simulink library "speedgoatlib_evse"  (R2024b)
settings: Solver=VariableStepAuto  StartTime=0.0  StopTime=10.0  RelTol=1e-3
undefined symbols (not defined in the file): sg_ev_charging_read_m, sg_ev_charging_write_m, sg_ev_isolation_read_m, sg_ev_parameter_read_m, sg_ev_parameter_write_m, sg_ev_precharge_read_m, sg_ev_precharge_write_m, sg_ev_status_m, sg_ev_stop_read_m, sg_ev_stop_write_m, sg_ev_welding_read_m, sg_ev_welding_write_m, sg_evse_charging_read_m, sg_evse_charging_write_m, sg_evse_isolation_read_m, sg_evse_isolation_write_m, sg_evse_parameter_read_m, sg_evse_parameter_write_m, sg_evse_precharge_read_m, sg_evse_precharge_write_m, sg_evse_status_m, sg_evse_stop_read_m, sg_evse_stop_write_m, sg_evse_welding_read_m, sg_evse_welding_write_m
libraries: speedgoatlib_mqtt x199, simulink x39, $bdroot x24
(part 5 of 8)

== system speedgoatlib_evse/Blocks by Charge State/EV Welding Read /string compare logic1 ==
  Input : Inport
  ASCII to String1 : ASCIIToString
  Add : Sum
  Gain : Gain  Gain=2
  String Compare : StringCompare
  String Compare1 : StringCompare
  String Constant : StringConstant  String="\"started\""
  String Constant1 : StringConstant  String="\"finished\""
  Out1 : Outport
  wires:
  Input/1 -> ASCII to String1/1
  Add/1 -> Out1/1
  Gain/1 -> Add/2
  String Compare1/1 -> Gain/1
  String Constant/1 -> String Compare/2
  String Compare/1 -> Add/1
  String Constant1/1 -> String Compare1/2
  ASCII to String1/1 -> String Compare/1, String Compare1/1

== system speedgoatlib_evse/Blocks by Charge State/EV Welding Write /Enabled Subsystem ==
  ready : Inport
  errorcode : Inport  Port=2
  resssoc : Inport  Port=3
  Enable : EnablePort
  Constant1 : Constant  Value=parEnErrorCode  OutDataTypeStr=boolean
  Constant2 : Constant  Value=parEnRessSoc  OutDataTypeStr=boolean
  Constant5 : Constant  Value=parEnReady  OutDataTypeStr=boolean
  Data Type Conversion1 : DataTypeConversion  OutDataTypeStr=double  SaturateOnIntegerOverflow=off  RndMeth=Floor
  Ground1 : Ground
  Ground2 : Ground
  Ground5 : Ground
  String to ASCII1 : StringToASCII  OutputVectorSize=12
  String to ASCII2 : StringToASCII  OutputVectorSize=12
  String to ASCII3 : StringToASCII  OutputVectorSize=24
  To String1 : ToString
  To String2 : ToString
  To String3 : ToString
  port0_ci_ev_welding_errorcode : speedgoatlib_mqtt/Client/MQTT Client Publish  ClientId=parClientId  ConnectionId=parConnectionId  Topic='port0/ci/ev/welding/errorcode'  QoS=0 - at most once  Retain=on  Extended=on  SampleTime=parSampleTime
      settings: SourceProductName=MQTT
  port0_ci_ev_welding_ready : speedgoatlib_mqtt/Client/MQTT Client Publish  ClientId=parClientId  ConnectionId=parConnectionId  Topic='port0/ci/ev/welding/ready'  QoS=0 - at most once  Retain=on  Extended=on  SampleTime=parSampleTime
      settings: SourceProductName=MQTT
  port0_ci_ev_welding_resssoc : speedgoatlib_mqtt/Client/MQTT Client Publish  ClientId=parClientId  ConnectionId=parConnectionId  Topic='port0/ci/ev/welding/resssoc'  QoS=0 - at most once  Retain=on  Extended=on  SampleTime=parSampleTime
      settings: SourceProductName=MQTT
  wires:
  ready/1 -> Data Type Conversion1/1
  To String1/1 -> String to ASCII1/1
  String to ASCII1/1 -> port0_ci_ev_welding_ready/1
  String to ASCII2/1 -> port0_ci_ev_welding_resssoc/1
  To String2/1 -> String to ASCII2/1
  resssoc/1 -> To String2/1
  Data Type Conversion1/1 -> To String1/1
  To String3/1 -> String to ASCII3/1
  errorcode/1 -> To String3/1
  String to ASCII3/1 -> port0_ci_ev_welding_errorcode/1
  Constant5/1 -> port0_ci_ev_welding_ready/2
  Ground5/1 -> port0_ci_ev_welding_ready/3
  Ground1/1 -> port0_ci_ev_welding_errorcode/3
  Constant1/1 -> port0_ci_ev_welding_errorcode/2
  Constant2/1 -> port0_ci_ev_welding_resssoc/2
  Ground2/1 -> port0_ci_ev_welding_resssoc/3

== system speedgoatlib_evse/Blocks by Charge State/EV Welding Write /string compare logic ==
  Input : Inport
  ASCII to String1 : ASCIIToString
  Add : Sum
  Gain : Gain  Gain=2
  String Compare : StringCompare
  String Compare1 : StringCompare
  String Constant : StringConstant  String="\"started\""
  String Constant1 : StringConstant  String="\"finished\""
  Out1 : Outport
  wires:
  ASCII to String1/1 -> String Compare1/1, String Compare/1
  String Constant1/1 -> String Compare1/2
  String Compare/1 -> Add/1
  String Constant/1 -> String Compare/2
  String Compare1/1 -> Gain/1
  Gain/1 -> Add/2
  Add/1 -> Out1/1
  Input/1 -> ASCII to String1/1

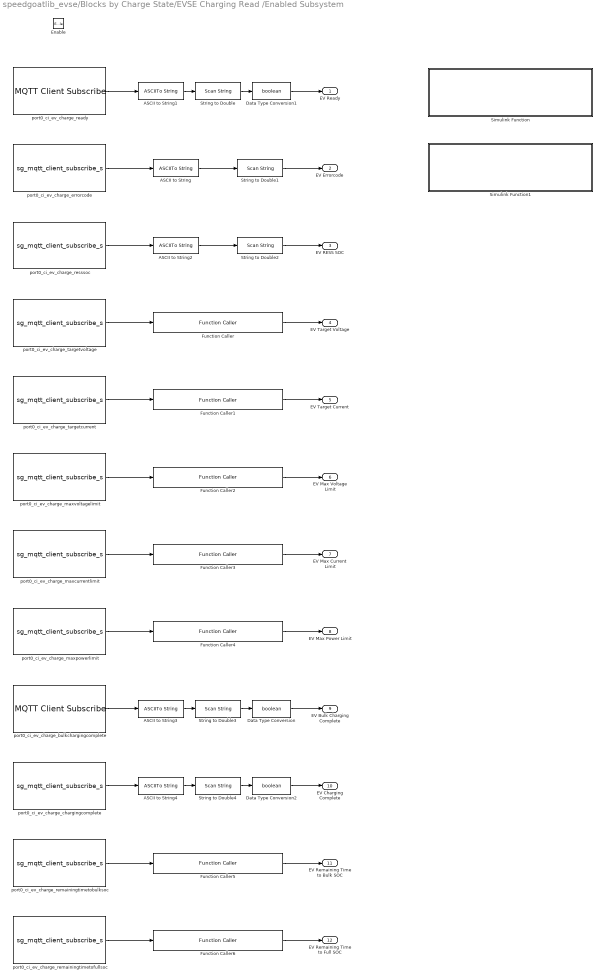
== system speedgoatlib_evse/Blocks by Charge State/EVSE Charging Read /Enabled Subsystem ==
  Enable : EnablePort
  ASCII to String{,1..4} (5 alike) : ASCIIToString
  Data Type Conversion : DataTypeConversion  OutDataTypeStr=boolean  SaturateOnIntegerOverflow=off  RndMeth=Floor
  Data Type Conversion1 : DataTypeConversion  OutDataTypeStr=boolean  SaturateOnIntegerOverflow=off  RndMeth=Floor
  Data Type Conversion2 : DataTypeConversion  OutDataTypeStr=boolean  SaturateOnIntegerOverflow=off  RndMeth=Floor
  Function Caller{,1..4} (5 alike) : FunctionCaller  FunctionPrototype=value = fromJsonPhysicalValue(uint8_vec)  InputArgumentSpecifications=zeros(1,48,'uint8')  OutputArgumentSpecifications=double(0)
  Function Caller5 : FunctionCaller  FunctionPrototype=value = fromJsonPhysicalValueUnit(uint8_vec)  InputArgumentSpecifications=zeros(1,64,'uint8')  OutputArgumentSpecifications=double(0)
  Function Caller6 : FunctionCaller  FunctionPrototype=value = fromJsonPhysicalValueUnit(uint8_vec)  InputArgumentSpecifications=zeros(1,64,'uint8')  OutputArgumentSpecifications=double(0)
  Simulink Function : Subsystem  TreatAsAtomicUnit=on
  Simulink Function1 : Subsystem  TreatAsAtomicUnit=on
  String to Double{,1..4} (5 alike) : ScanString  Format="\"%lf\""
  port0_ci_ev_charge_bulkchargingcomplete : speedgoatlib_mqtt/Client/MQTT Client Subscribe  ClientId=parClientId  ConnectionId=parConnectionId  Topic='port0/ci/ev/charge/bulkchargingcomplete'  QoS=0 - at most once  InitValue=zeros(1,12,'uint8')  Extended=off  SampleTime=parSampleTime
      settings: SourceProductName=MQTT
  port0_ci_ev_charge_chargingcomplete : S-Function  FunctionName=sg_mqtt_client_subscribe_s  Parameters="ClientId,  ConnectionId, Topic, QoS, InitValue, Extended, SampleTime"  SFunctionDeploymentMode=off  EnableBusSupport=off  mask(mqtt_client_subscribe_1){ClientId=parClientId, ConnectionId=parConnectionId, Topic='port0/ci/ev/charge/chargingcomplete', QoS=0 - at most once, InitValue=zeros(1,12,'uint8'), Extended=off, SampleTime=parSampleTime}
      mask prompts: ClientId "Station ID"; ConnectionId "Connection ID"; QoS "Quality of Service"; InitValue "Init Value"; Extended "Extended Interface"; SampleTime "Sample Time [s]"
      mask help: Speedgoat Driver Block<br>MQTT Client - Subscribe<br><br>&copy; 2007 - 2023, Speedgoat GmbH, <a href="matlab: web('www.speedgoat.com','-browser');">www.speedgoat.com</a>
      mask init:
      | sg_mqtt_client_subscribe_m.runMaskInitialization(ClientId, ConnectionId, Topic, InitValue, Extended);
      mask Help: eval('sg.utils.help.show(''io_main/refentry_mqtt_client_subscribe'');')
      mask TypeOptions QoS: 0 - at most once | 1 - at least once | 2 - exactly once
      mask DialogControl groupParameters Prompt: Parameters
      mask Display: disp('Speedgoat\nMQTT Client\nSubscribe\nStation ID: 0\nConnection ID: 0');
  port0_ci_ev_charge_errorcode : S-Function  FunctionName=sg_mqtt_client_subscribe_s  Parameters="ClientId,  ConnectionId, Topic, QoS, InitValue, Extended, SampleTime"  SFunctionDeploymentMode=off  EnableBusSupport=off  mask(mqtt_client_subscribe_1){ClientId=parClientId, ConnectionId=parConnectionId, Topic='port0/ci/ev/charge/errorcode', QoS=0 - at most once, InitValue=zeros(1,24,'uint8'), Extended=off, SampleTime=parSampleTime}
      mask prompts: ClientId "Station ID"; ConnectionId "Connection ID"; QoS "Quality of Service"; InitValue "Init Value"; Extended "Extended Interface"; SampleTime "Sample Time [s]"
      mask help: Speedgoat Driver Block<br>MQTT Client - Subscribe<br><br>&copy; 2007 - 2023, Speedgoat GmbH, <a href="matlab: web('www.speedgoat.com','-browser');">www.speedgoat.com</a>
      mask init:
      | sg_mqtt_client_subscribe_m.runMaskInitialization(ClientId, ConnectionId, Topic, InitValue, Extended);
      mask Help: eval('sg.utils.help.show(''io_main/refentry_mqtt_client_subscribe'');')
      mask TypeOptions QoS: 0 - at most once | 1 - at least once | 2 - exactly once
      mask DialogControl groupParameters Prompt: Parameters
      mask Display: disp('Speedgoat\nMQTT Client\nSubscribe\nStation ID: 0\nConnection ID: 0');
  port0_ci_ev_charge_maxcurrentlimit : S-Function  FunctionName=sg_mqtt_client_subscribe_s  Parameters="ClientId,  ConnectionId, Topic, QoS, InitValue, Extended, SampleTime"  SFunctionDeploymentMode=off  EnableBusSupport=off  mask(mqtt_client_subscribe_1){ClientId=parClientId, ConnectionId=parConnectionId, Topic='port0/ci/ev/charge/maxcurrentlimit', QoS=0 - at most once, InitValue=zeros(1,48,'uint8'), Extended=off, SampleTime=parSampleTime}
      mask prompts: ClientId "Station ID"; ConnectionId "Connection ID"; QoS "Quality of Service"; InitValue "Init Value"; Extended "Extended Interface"; SampleTime "Sample Time [s]"
      mask help: Speedgoat Driver Block<br>MQTT Client - Subscribe<br><br>&copy; 2007 - 2023, Speedgoat GmbH, <a href="matlab: web('www.speedgoat.com','-browser');">www.speedgoat.com</a>
      mask init:
      | sg_mqtt_client_subscribe_m.runMaskInitialization(ClientId, ConnectionId, Topic, InitValue, Extended);
      mask Help: eval('sg.utils.help.show(''io_main/refentry_mqtt_client_subscribe'');')
      mask TypeOptions QoS: 0 - at most once | 1 - at least once | 2 - exactly once
      mask DialogControl groupParameters Prompt: Parameters
      mask Display: disp('Speedgoat\nMQTT Client\nSubscribe\nStation ID: 0\nConnection ID: 0');
  port0_ci_ev_charge_maxpowerlimit : S-Function  FunctionName=sg_mqtt_client_subscribe_s  Parameters="ClientId,  ConnectionId, Topic, QoS, InitValue, Extended, SampleTime"  SFunctionDeploymentMode=off  EnableBusSupport=off  mask(mqtt_client_subscribe_1){ClientId=parClientId, ConnectionId=parConnectionId, Topic='port0/ci/ev/charge/maxpowerlimit', QoS=0 - at most once, InitValue=zeros(1,48,'uint8'), Extended=off, SampleTime=parSampleTime}
      mask prompts: ClientId "Station ID"; ConnectionId "Connection ID"; QoS "Quality of Service"; InitValue "Init Value"; Extended "Extended Interface"; SampleTime "Sample Time [s]"
      mask help: Speedgoat Driver Block<br>MQTT Client - Subscribe<br><br>&copy; 2007 - 2023, Speedgoat GmbH, <a href="matlab: web('www.speedgoat.com','-browser');">www.speedgoat.com</a>
      mask init:
      | sg_mqtt_client_subscribe_m.runMaskInitialization(ClientId, ConnectionId, Topic, InitValue, Extended);
      mask Help: eval('sg.utils.help.show(''io_main/refentry_mqtt_client_subscribe'');')
      mask TypeOptions QoS: 0 - at most once | 1 - at least once | 2 - exactly once
      mask DialogControl groupParameters Prompt: Parameters
      mask Display: disp('Speedgoat\nMQTT Client\nSubscribe\nStation ID: 0\nConnection ID: 0');
  port0_ci_ev_charge_maxvoltagelimit : S-Function  FunctionName=sg_mqtt_client_subscribe_s  Parameters="ClientId,  ConnectionId, Topic, QoS, InitValue, Extended, SampleTime"  SFunctionDeploymentMode=off  EnableBusSupport=off  mask(mqtt_client_subscribe_1){ClientId=parClientId, ConnectionId=parConnectionId, Topic='port0/ci/ev/charge/maxvoltagelimit', QoS=0 - at most once, InitValue=zeros(1,48,'uint8'), Extended=off, SampleTime=parSampleTime}
      mask prompts: ClientId "Station ID"; ConnectionId "Connection ID"; QoS "Quality of Service"; InitValue "Init Value"; Extended "Extended Interface"; SampleTime "Sample Time [s]"
      mask help: Speedgoat Driver Block<br>MQTT Client - Subscribe<br><br>&copy; 2007 - 2023, Speedgoat GmbH, <a href="matlab: web('www.speedgoat.com','-browser');">www.speedgoat.com</a>
      mask init:
      | sg_mqtt_client_subscribe_m.runMaskInitialization(ClientId, ConnectionId, Topic, InitValue, Extended);
      mask Help: eval('sg.utils.help.show(''io_main/refentry_mqtt_client_subscribe'');')
      mask TypeOptions QoS: 0 - at most once | 1 - at least once | 2 - exactly once
      mask DialogControl groupParameters Prompt: Parameters
      mask Display: disp('Speedgoat\nMQTT Client\nSubscribe\nStation ID: 0\nConnection ID: 0');
  port0_ci_ev_charge_ready : speedgoatlib_mqtt/Client/MQTT Client Subscribe  ClientId=parClientId  ConnectionId=parConnectionId  Topic='port0/ci/ev/charge/ready'  QoS=0 - at most once  InitValue=zeros(1,12,'uint8')  Extended=off  SampleTime=parSampleTime
      settings: SourceProductName=MQTT
  port0_ci_ev_charge_remainingtimetobulksoc : S-Function  FunctionName=sg_mqtt_client_subscribe_s  Parameters="ClientId,  ConnectionId, Topic, QoS, InitValue, Extended, SampleTime"  SFunctionDeploymentMode=off  EnableBusSupport=off  mask(mqtt_client_subscribe_1){ClientId=parClientId, ConnectionId=parConnectionId, Topic='port0/ci/ev/charge/remainingtimetobulksoc', QoS=0 - at most once, InitValue=zeros(1,64,'uint8'), Extended=off, SampleTime=parSampleTime}
      mask prompts: ClientId "Station ID"; ConnectionId "Connection ID"; QoS "Quality of Service"; InitValue "Init Value"; Extended "Extended Interface"; SampleTime "Sample Time [s]"
      mask help: Speedgoat Driver Block<br>MQTT Client - Subscribe<br><br>&copy; 2007 - 2023, Speedgoat GmbH, <a href="matlab: web('www.speedgoat.com','-browser');">www.speedgoat.com</a>
      mask init:
      | sg_mqtt_client_subscribe_m.runMaskInitialization(ClientId, ConnectionId, Topic, InitValue, Extended);
      mask Help: eval('sg.utils.help.show(''io_main/refentry_mqtt_client_subscribe'');')
      mask TypeOptions QoS: 0 - at most once | 1 - at least once | 2 - exactly once
      mask DialogControl groupParameters Prompt: Parameters
      mask Display: disp('Speedgoat\nMQTT Client\nSubscribe\nStation ID: 0\nConnection ID: 0');
  port0_ci_ev_charge_remainingtimetofullsoc : S-Function  FunctionName=sg_mqtt_client_subscribe_s  Parameters="ClientId,  ConnectionId, Topic, QoS, InitValue, Extended, SampleTime"  SFunctionDeploymentMode=off  EnableBusSupport=off  mask(mqtt_client_subscribe_1){ClientId=parClientId, ConnectionId=parConnectionId, Topic='port0/ci/ev/charge/remainingtimetofullsoc', QoS=0 - at most once, InitValue=zeros(1,64,'uint8'), Extended=off, SampleTime=parSampleTime}
      mask prompts: ClientId "Station ID"; ConnectionId "Connection ID"; QoS "Quality of Service"; InitValue "Init Value"; Extended "Extended Interface"; SampleTime "Sample Time [s]"
      mask help: Speedgoat Driver Block<br>MQTT Client - Subscribe<br><br>&copy; 2007 - 2023, Speedgoat GmbH, <a href="matlab: web('www.speedgoat.com','-browser');">www.speedgoat.com</a>
      mask init:
      | sg_mqtt_client_subscribe_m.runMaskInitialization(ClientId, ConnectionId, Topic, InitValue, Extended);
      mask Help: eval('sg.utils.help.show(''io_main/refentry_mqtt_client_subscribe'');')
      mask TypeOptions QoS: 0 - at most once | 1 - at least once | 2 - exactly once
      mask DialogControl groupParameters Prompt: Parameters
      mask Display: disp('Speedgoat\nMQTT Client\nSubscribe\nStation ID: 0\nConnection ID: 0');
  port0_ci_ev_charge_resssoc : S-Function  FunctionName=sg_mqtt_client_subscribe_s  Parameters="ClientId,  ConnectionId, Topic, QoS, InitValue, Extended, SampleTime"  SFunctionDeploymentMode=off  EnableBusSupport=off  mask(mqtt_client_subscribe_1){ClientId=parClientId, ConnectionId=parConnectionId, Topic='port0/ci/ev/charge/resssoc', QoS=0 - at most once, InitValue=zeros(1,12,'uint8'), Extended=off, SampleTime=parSampleTime}
      mask prompts: ClientId "Station ID"; ConnectionId "Connection ID"; QoS "Quality of Service"; InitValue "Init Value"; Extended "Extended Interface"; SampleTime "Sample Time [s]"
      mask help: Speedgoat Driver Block<br>MQTT Client - Subscribe<br><br>&copy; 2007 - 2023, Speedgoat GmbH, <a href="matlab: web('www.speedgoat.com','-browser');">www.speedgoat.com</a>
      mask init:
      | sg_mqtt_client_subscribe_m.runMaskInitialization(ClientId, ConnectionId, Topic, InitValue, Extended);
      mask Help: eval('sg.utils.help.show(''io_main/refentry_mqtt_client_subscribe'');')
      mask TypeOptions QoS: 0 - at most once | 1 - at least once | 2 - exactly once
      mask DialogControl groupParameters Prompt: Parameters
      mask Display: disp('Speedgoat\nMQTT Client\nSubscribe\nStation ID: 0\nConnection ID: 0');
  port0_ci_ev_charge_targetcurrent : S-Function  FunctionName=sg_mqtt_client_subscribe_s  Parameters="ClientId,  ConnectionId, Topic, QoS, InitValue, Extended, SampleTime"  SFunctionDeploymentMode=off  EnableBusSupport=off  mask(mqtt_client_subscribe_1){ClientId=parClientId, ConnectionId=parConnectionId, Topic='port0/ci/ev/charge/targetcurrent', QoS=0 - at most once, InitValue=zeros(1,48,'uint8'), Extended=off, SampleTime=parSampleTime}
      mask prompts: ClientId "Station ID"; ConnectionId "Connection ID"; QoS "Quality of Service"; InitValue "Init Value"; Extended "Extended Interface"; SampleTime "Sample Time [s]"
      mask help: Speedgoat Driver Block<br>MQTT Client - Subscribe<br><br>&copy; 2007 - 2023, Speedgoat GmbH, <a href="matlab: web('www.speedgoat.com','-browser');">www.speedgoat.com</a>
      mask init:
      | sg_mqtt_client_subscribe_m.runMaskInitialization(ClientId, ConnectionId, Topic, InitValue, Extended);
      mask Help: eval('sg.utils.help.show(''io_main/refentry_mqtt_client_subscribe'');')
      mask TypeOptions QoS: 0 - at most once | 1 - at least once | 2 - exactly once
      mask DialogControl groupParameters Prompt: Parameters
      mask Display: disp('Speedgoat\nMQTT Client\nSubscribe\nStation ID: 0\nConnection ID: 0');
  port0_ci_ev_charge_targetvoltage : S-Function  FunctionName=sg_mqtt_client_subscribe_s  Parameters="ClientId,  ConnectionId, Topic, QoS, InitValue, Extended, SampleTime"  SFunctionDeploymentMode=off  EnableBusSupport=off  mask(mqtt_client_subscribe_1){ClientId=parClientId, ConnectionId=parConnectionId, Topic='port0/ci/ev/charge/targetvoltage', QoS=0 - at most once, InitValue=zeros(1,48,'uint8'), Extended=off, SampleTime=parSampleTime}
      mask prompts: ClientId "Station ID"; ConnectionId "Connection ID"; QoS "Quality of Service"; InitValue "Init Value"; Extended "Extended Interface"; SampleTime "Sample Time [s]"
      mask help: Speedgoat Driver Block<br>MQTT Client - Subscribe<br><br>&copy; 2007 - 2023, Speedgoat GmbH, <a href="matlab: web('www.speedgoat.com','-browser');">www.speedgoat.com</a>
      mask init:
      | sg_mqtt_client_subscribe_m.runMaskInitialization(ClientId, ConnectionId, Topic, InitValue, Extended);
      mask Help: eval('sg.utils.help.show(''io_main/refentry_mqtt_client_subscribe'');')
      mask TypeOptions QoS: 0 - at most once | 1 - at least once | 2 - exactly once
      mask DialogControl groupParameters Prompt: Parameters
      mask Display: disp('Speedgoat\nMQTT Client\nSubscribe\nStation ID: 0\nConnection ID: 0');
  EV Ready : Outport
  EV Errorcode : Outport  Port=2
  EV RESS SOC : Outport  Port=3
  EV Target Voltage : Outport  Port=4
  EV Target Current : Outport  Port=5
  EV Max Voltage Limit : Outport  Port=6
  EV Max Current Limit : Outport  Port=7
  EV Max Power Limit : Outport  Port=8
  EV Bulk Charging Complete : Outport  Port=9
  EV Charging Complete : Outport  Port=10
  EV Remaining Time to Bulk SOC : Outport  Port=11
  EV Remaining Time to Full SOC : Outport  Port=12
  wires:
  port0_ci_ev_charge_ready/1 -> ASCII to String1/1
  port0_ci_ev_charge_errorcode/1 -> ASCII to String/1
  ASCII to String/1 -> String to Double1/1
  ASCII to String1/1 -> String to Double/1
  String to Double/1 -> Data Type Conversion1/1
  String to Double1/1 -> EV Errorcode/1
  String to Double2/1 -> EV RESS SOC/1
  ASCII to String2/1 -> String to Double2/1
  port0_ci_ev_charge_resssoc/1 -> ASCII to String2/1
  Function Caller/1 -> EV Target Voltage/1
  port0_ci_ev_charge_targetvoltage/1 -> Function Caller/1
  port0_ci_ev_charge_targetcurrent/1 -> Function Caller1/1
  Function Caller1/1 -> EV Target Current/1
  Function Caller2/1 -> EV Max Voltage Limit/1
  port0_ci_ev_charge_maxvoltagelimit/1 -> Function Caller2/1
  port0_ci_ev_charge_maxcurrentlimit/1 -> Function Caller3/1
  Function Caller3/1 -> EV Max Current Limit/1
  Function Caller4/1 -> EV Max Power Limit/1
  port0_ci_ev_charge_maxpowerlimit/1 -> Function Caller4/1
  String to Double3/1 -> Data Type Conversion/1
  ASCII to String3/1 -> String to Double3/1
  port0_ci_ev_charge_bulkchargingcomplete/1 -> ASCII to String3/1
  Data Type Conversion/1 -> EV Bulk Charging Complete/1
  Data Type Conversion1/1 -> EV Ready/1
  Data Type Conversion2/1 -> EV Charging Complete/1
  port0_ci_ev_charge_chargingcomplete/1 -> ASCII to String4/1
  ASCII to String4/1 -> String to Double4/1
  String to Double4/1 -> Data Type Conversion2/1
  port0_ci_ev_charge_remainingtimetobulksoc/1 -> Function Caller5/1
  Function Caller5/1 -> EV Remaining Time to Bulk SOC/1
  Function Caller6/1 -> EV Remaining Time to Full SOC/1
  port0_ci_ev_charge_remainingtimetofullsoc/1 -> Function Caller6/1

== system speedgoatlib_evse/Blocks by Charge State/EVSE Charging Read /string compare logic ==
  Input : Inport
  ASCII to String1 : ASCIIToString
  Add : Sum
  Gain : Gain  Gain=2
  String Compare : StringCompare
  String Compare1 : StringCompare
  String Constant : StringConstant  String="\"started\""
  String Constant1 : StringConstant  String="\"finished\""
  Out1 : Outport
  wires:
  Input/1 -> ASCII to String1/1
  Add/1 -> Out1/1
  Gain/1 -> Add/2
  String Compare1/1 -> Gain/1
  String Constant/1 -> String Compare/2
  String Compare/1 -> Add/1
  String Constant1/1 -> String Compare1/2
  ASCII to String1/1 -> String Compare/1, String Compare1/1

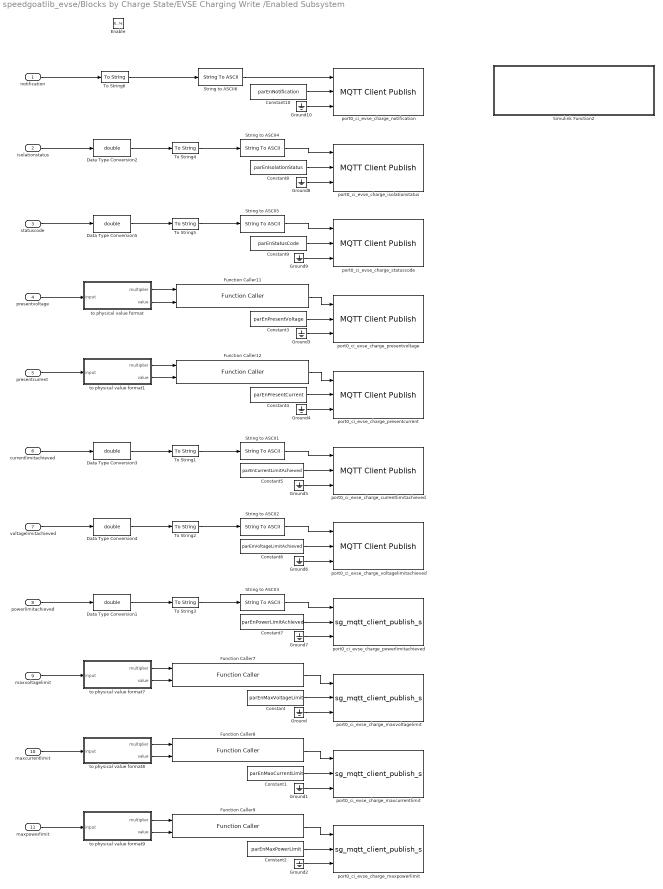
== system speedgoatlib_evse/Blocks by Charge State/EVSE Charging Write /Enabled Subsystem ==
  notification : Inport
  isolationstatus : Inport  Port=2
  statuscode : Inport  Port=3
  presentvoltage : Inport  Port=4
  presentcurrent : Inport  Port=5
  currentlimitachieved : Inport  Port=6
  voltagelimitachieved : Inport  Port=7
  powerlimitachieved : Inport  Port=8
  maxvoltagelimit : Inport  Port=9
  maxcurrentlimit : Inport  Port=10
  maxpowerlimit : Inport  Port=11
  Enable : EnablePort
  Constant : Constant  Value=parEnMaxVoltageLimit  OutDataTypeStr=boolean
  Constant1 : Constant  Value=parEnMaxCurrentLimit  OutDataTypeStr=boolean
  Constant10 : Constant  Value=parEnNotification  OutDataTypeStr=boolean
  Constant2 : Constant  Value=parEnMaxPowerLimit  OutDataTypeStr=boolean
  Constant3 : Constant  Value=parEnPresentVoltage  OutDataTypeStr=boolean
  Constant4 : Constant  Value=parEnPresentCurrent  OutDataTypeStr=boolean
  Constant5 : Constant  Value=parEnCurrentLimitAchieved  OutDataTypeStr=boolean
  Constant6 : Constant  Value=parEnVoltageLimitAchieved  OutDataTypeStr=boolean
  Constant7 : Constant  Value=parEnPowerLimitAchieved  OutDataTypeStr=boolean
  Constant8 : Constant  Value=parEnIsolationStatus  OutDataTypeStr=boolean
  Constant9 : Constant  Value=parEnStatusCode  OutDataTypeStr=boolean
  Data Type Conversion{1..5} (5 alike) : DataTypeConversion  OutDataTypeStr=double  SaturateOnIntegerOverflow=off  RndMeth=Floor
  Function Caller{7..9,11..12} (5 alike) : FunctionCaller  FunctionPrototype=json_string = toJsonPhysicalValue(multiplier,value)  InputArgumentSpecifications=double(0), double(0)  OutputArgumentSpecifications=zeros(1,48,'uint8')
  Ground{,1..10} (11 alike) : Ground
  Simulink Function2 : Subsystem  TreatAsAtomicUnit=on
  String to ASCII{1..5} (5 alike) : StringToASCII  OutputVectorSize=12
  String to ASCII6 : StringToASCII  OutputVectorSize=16
  To String{1..6} (6 alike) : ToString
  port0_ci_evse_charge_currentlimitachieved : speedgoatlib_mqtt/Client/MQTT Client Publish  ClientId=parClientId  ConnectionId=parConnectionId  Topic='port0/ci/evse/charge/currentlimitachieved'  QoS=0 - at most once  Retain=on  Extended=on  SampleTime=parSampleTime
      settings: SourceProductName=MQTT
  port0_ci_evse_charge_isolationstatus : speedgoatlib_mqtt/Client/MQTT Client Publish  ClientId=parClientId  ConnectionId=parConnectionId  Topic='port0/ci/evse/charge/isolationstatus'  QoS=0 - at most once  Retain=on  Extended=on  SampleTime=parSampleTime
      settings: SourceProductName=MQTT
  port0_ci_evse_charge_maxcurrentlimit : S-Function  FunctionName=sg_mqtt_client_publish_s  Parameters="ClientId,  ConnectionId, Topic, QoS, Retain, Extended, SampleTime"  SFunctionDeploymentMode=off  EnableBusSupport=off  mask(mqtt_client_publish_1){ClientId=parClientId, ConnectionId=parConnectionId, Topic='port0/ci/evse/charge/maxcurrentlimit', QoS=0 - at most once, Retain=on, Extended=on, SampleTime=parSampleTime}
      mask prompts: ClientId "Station ID"; ConnectionId "Connection ID"; QoS "Quality of Service"; Extended "Extended Interface"; SampleTime "Sample Time [s]"
      mask help: Speedgoat Driver Block<br>MQTT Client - Publish<br><br>&copy; 2007 - 2023, Speedgoat GmbH, <a href="matlab: web('www.speedgoat.com','-browser');">www.speedgoat.com</a>
      mask init:
      | sg_mqtt_client_publish_m.runMaskInitialization(ClientId, ConnectionId, Topic, Extended);
      mask Help: eval('sg.utils.help.show(''io_main/refentry_mqtt_client_publish'');')
      mask TypeOptions QoS: 0 - at most once | 1 - at least once | 2 - exactly once
      mask DialogControl groupParameters Prompt: Parameters
      mask Display: text(0.9,0.5,'Speedgoat\nMQTT Client\nPublish\nStation ID: 0\nConnection ID: 0','horizontalAlignment', 'right','verticalAlignment', 'middle');port_label('input',1,'Data');port_label('input',2,'Enable');port_label('input',3,'Length');
  port0_ci_evse_charge_maxpowerlimit : S-Function  FunctionName=sg_mqtt_client_publish_s  Parameters="ClientId,  ConnectionId, Topic, QoS, Retain, Extended, SampleTime"  SFunctionDeploymentMode=off  EnableBusSupport=off  mask(mqtt_client_publish_1){ClientId=parClientId, ConnectionId=parConnectionId, Topic='port0/ci/evse/charge/maxpowerlimit', QoS=0 - at most once, Retain=on, Extended=on, SampleTime=parSampleTime}
      mask prompts: ClientId "Station ID"; ConnectionId "Connection ID"; QoS "Quality of Service"; Extended "Extended Interface"; SampleTime "Sample Time [s]"
      mask help: Speedgoat Driver Block<br>MQTT Client - Publish<br><br>&copy; 2007 - 2023, Speedgoat GmbH, <a href="matlab: web('www.speedgoat.com','-browser');">www.speedgoat.com</a>
      mask init:
      | sg_mqtt_client_publish_m.runMaskInitialization(ClientId, ConnectionId, Topic, Extended);
      mask Help: eval('sg.utils.help.show(''io_main/refentry_mqtt_client_publish'');')
      mask TypeOptions QoS: 0 - at most once | 1 - at least once | 2 - exactly once
      mask DialogControl groupParameters Prompt: Parameters
      mask Display: text(0.9,0.5,'Speedgoat\nMQTT Client\nPublish\nStation ID: 0\nConnection ID: 0','horizontalAlignment', 'right','verticalAlignment', 'middle');port_label('input',1,'Data');port_label('input',2,'Enable');port_label('input',3,'Length');
  port0_ci_evse_charge_maxvoltagelimit : S-Function  FunctionName=sg_mqtt_client_publish_s  Parameters="ClientId,  ConnectionId, Topic, QoS, Retain, Extended, SampleTime"  SFunctionDeploymentMode=off  EnableBusSupport=off  mask(mqtt_client_publish_1){ClientId=parClientId, ConnectionId=parConnectionId, Topic='port0/ci/evse/charge/maxvoltagelimit', QoS=0 - at most once, Retain=on, Extended=on, SampleTime=parSampleTime}
      mask prompts: ClientId "Station ID"; ConnectionId "Connection ID"; QoS "Quality of Service"; Extended "Extended Interface"; SampleTime "Sample Time [s]"
      mask help: Speedgoat Driver Block<br>MQTT Client - Publish<br><br>&copy; 2007 - 2023, Speedgoat GmbH, <a href="matlab: web('www.speedgoat.com','-browser');">www.speedgoat.com</a>
      mask init:
      | sg_mqtt_client_publish_m.runMaskInitialization(ClientId, ConnectionId, Topic, Extended);
      mask Help: eval('sg.utils.help.show(''io_main/refentry_mqtt_client_publish'');')
      mask TypeOptions QoS: 0 - at most once | 1 - at least once | 2 - exactly once
      mask DialogControl groupParameters Prompt: Parameters
      mask Display: text(0.9,0.5,'Speedgoat\nMQTT Client\nPublish\nStation ID: 0\nConnection ID: 0','horizontalAlignment', 'right','verticalAlignment', 'middle');port_label('input',1,'Data');port_label('input',2,'Enable');port_label('input',3,'Length');
  port0_ci_evse_charge_notification : speedgoatlib_mqtt/Client/MQTT Client Publish  ClientId=parClientId  ConnectionId=parConnectionId  Topic='port0/ci/evse/charge/notification'  QoS=0 - at most once  Retain=on  Extended=on  SampleTime=parSampleTime
      settings: SourceProductName=MQTT
  port0_ci_evse_charge_powerlimitachieved : S-Function  FunctionName=sg_mqtt_client_publish_s  Parameters="ClientId,  ConnectionId, Topic, QoS, Retain, Extended, SampleTime"  SFunctionDeploymentMode=off  EnableBusSupport=off  mask(mqtt_client_publish_1){ClientId=parClientId, ConnectionId=parConnectionId, Topic='port0/ci/evse/charge/powerlimitachieved', QoS=0 - at most once, Retain=on, Extended=on, SampleTime=parSampleTime}
      mask prompts: ClientId "Station ID"; ConnectionId "Connection ID"; QoS "Quality of Service"; Extended "Extended Interface"; SampleTime "Sample Time [s]"
      mask help: Speedgoat Driver Block<br>MQTT Client - Publish<br><br>&copy; 2007 - 2023, Speedgoat GmbH, <a href="matlab: web('www.speedgoat.com','-browser');">www.speedgoat.com</a>
      mask init:
      | sg_mqtt_client_publish_m.runMaskInitialization(ClientId, ConnectionId, Topic, Extended);
      mask Help: eval('sg.utils.help.show(''io_main/refentry_mqtt_client_publish'');')
      mask TypeOptions QoS: 0 - at most once | 1 - at least once | 2 - exactly once
      mask DialogControl groupParameters Prompt: Parameters
      mask Display: text(0.9,0.5,'Speedgoat\nMQTT Client\nPublish\nStation ID: 0\nConnection ID: 0','horizontalAlignment', 'right','verticalAlignment', 'middle');port_label('input',1,'Data');port_label('input',2,'Enable');port_label('input',3,'Length');
  port0_ci_evse_charge_presentcurrent : speedgoatlib_mqtt/Client/MQTT Client Publish  ClientId=parClientId  ConnectionId=parConnectionId  Topic='port0/ci/evse/charge/presentcurrent'  QoS=0 - at most once  Retain=on  Extended=on  SampleTime=parSampleTime
      settings: SourceProductName=MQTT
  port0_ci_evse_charge_presentvoltage : speedgoatlib_mqtt/Client/MQTT Client Publish  ClientId=parClientId  ConnectionId=parConnectionId  Topic='port0/ci/evse/charge/presentvoltage'  QoS=0 - at most once  Retain=on  Extended=on  SampleTime=parSampleTime
      settings: SourceProductName=MQTT
  port0_ci_evse_charge_statuscode : speedgoatlib_mqtt/Client/MQTT Client Publish  ClientId=parClientId  ConnectionId=parConnectionId  Topic='port0/ci/evse/charge/statuscode'  QoS=0 - at most once  Retain=on  Extended=on  SampleTime=parSampleTime
      settings: SourceProductName=MQTT
  port0_ci_evse_charge_voltagelimitachieved : speedgoatlib_mqtt/Client/MQTT Client Publish  ClientId=parClientId  ConnectionId=parConnectionId  Topic='port0/ci/evse/charge/voltagelimitachieved'  QoS=0 - at most once  Retain=on  Extended=on  SampleTime=parSampleTime
      settings: SourceProductName=MQTT
  to physical value format : MATLAB Function  TreatAsAtomicUnit=on
  to physical value format1 : MATLAB Function  TreatAsAtomicUnit=on
  to physical value format7 : MATLAB Function  TreatAsAtomicUnit=on
  to physical value format8 : MATLAB Function  TreatAsAtomicUnit=on
  to physical value format9 : MATLAB Function  TreatAsAtomicUnit=on
  wires:
  to physical value format1/2(value) -> Function Caller12/2
  to physical value format1/1(multiplier) -> Function Caller12/1
  to physical value format/2(value) -> Function Caller11/2
  to physical value format/1(multiplier) -> Function Caller11/1
  Function Caller12/1 -> port0_ci_evse_charge_presentcurrent/1
  Function Caller11/1 -> port0_ci_evse_charge_presentvoltage/1
  to physical value format9/1(multiplier) -> Function Caller9/1
  to physical value format9/2(value) -> Function Caller9/2
  Ground2/1 -> port0_ci_evse_charge_maxpowerlimit/3
  Constant2/1 -> port0_ci_evse_charge_maxpowerlimit/2
  Function Caller9/1 -> port0_ci_evse_charge_maxpowerlimit/1
  to physical value format8/2(value) -> Function Caller8/2
  to physical value format8/1(multiplier) -> Function Caller8/1
  Ground1/1 -> port0_ci_evse_charge_maxcurrentlimit/3
  Constant1/1 -> port0_ci_evse_charge_maxcurrentlimit/2
  Function Caller8/1 -> port0_ci_evse_charge_maxcurrentlimit/1
  to physical value format7/2(value) -> Function Caller7/2
  Function Caller7/1 -> port0_ci_evse_charge_maxvoltagelimit/1
  to physical value format7/1(multiplier) -> Function Caller7/1
  Ground/1 -> port0_ci_evse_charge_maxvoltagelimit/3
  Constant/1 -> port0_ci_evse_charge_maxvoltagelimit/2
  Data Type Conversion4/1 -> To String2/1
  To String2/1 -> String to ASCII2/1
  To String1/1 -> String to ASCII1/1
  Data Type Conversion3/1 -> To String1/1
  String to ASCII1/1 -> port0_ci_evse_charge_currentlimitachieved/1
  String to ASCII2/1 -> port0_ci_evse_charge_voltagelimitachieved/1
  presentvoltage/1 -> to physical value format/1(input)
  presentcurrent/1 -> to physical value format1/1(input)
  currentlimitachieved/1 -> Data Type Conversion3/1
  voltagelimitachieved/1 -> Data Type Conversion4/1
  maxvoltagelimit/1 -> to physical value format7/1(input)
  maxcurrentlimit/1 -> to physical value format8/1(input)
  maxpowerlimit/1 -> to physical value format9/1(input)
  powerlimitachieved/1 -> Data Type Conversion1/1
  String to ASCII3/1 -> port0_ci_evse_charge_powerlimitachieved/1
  To String3/1 -> String to ASCII3/1
  Data Type Conversion1/1 -> To String3/1
  Constant3/1 -> port0_ci_evse_charge_presentvoltage/2
  Ground3/1 -> port0_ci_evse_charge_presentvoltage/3
  Ground4/1 -> port0_ci_evse_charge_presentcurrent/3
  Constant4/1 -> port0_ci_evse_charge_presentcurrent/2
  Constant5/1 -> port0_ci_evse_charge_currentlimitachieved/2
  Ground5/1 -> port0_ci_evse_charge_currentlimitachieved/3
  Constant6/1 -> port0_ci_evse_charge_voltagelimitachieved/2
  Ground6/1 -> port0_ci_evse_charge_voltagelimitachieved/3
  Ground7/1 -> port0_ci_evse_charge_powerlimitachieved/3
  Constant7/1 -> port0_ci_evse_charge_powerlimitachieved/2
  Ground10/1 -> port0_ci_evse_charge_notification/3
  String to ASCII6/1 -> port0_ci_evse_charge_notification/1
  Constant10/1 -> port0_ci_evse_charge_notification/2
  To String6/1 -> String to ASCII6/1
  String to ASCII4/1 -> port0_ci_evse_charge_isolationstatus/1
  isolationstatus/1 -> Data Type Conversion2/1
  Data Type Conversion2/1 -> To String4/1
  Constant9/1 -> port0_ci_evse_charge_statuscode/2
  statuscode/1 -> Data Type Conversion5/1
  Ground9/1 -> port0_ci_evse_charge_statuscode/3
  Data Type Conversion5/1 -> To String5/1
  To String5/1 -> String to ASCII5/1
  Ground8/1 -> port0_ci_evse_charge_isolationstatus/3
  Constant8/1 -> port0_ci_evse_charge_isolationstatus/2
  To String4/1 -> String to ASCII4/1
  notification/1 -> To String6/1
  String to ASCII5/1 -> port0_ci_evse_charge_statuscode/1

== system speedgoatlib_evse/Blocks by Charge State/EVSE Charging Write /string compare logic ==
  Input : Inport
  ASCII to String1 : ASCIIToString
  Add : Sum
  Gain : Gain  Gain=2
  String Compare : StringCompare
  String Compare1 : StringCompare
  String Constant : StringConstant  String="\"started\""
  String Constant1 : StringConstant  String="\"finished\""
  Out1 : Outport
  wires:
  ASCII to String1/1 -> String Compare1/1, String Compare/1
  String Constant1/1 -> String Compare1/2
  String Compare/1 -> Add/1
  String Constant/1 -> String Compare/2
  String Compare1/1 -> Gain/1
  Gain/1 -> Add/2
  Add/1 -> Out1/1
  Input/1 -> ASCII to String1/1

== system speedgoatlib_evse/Blocks by Charge State/EVSE Isolation Read /Enabled Subsystem ==
  Enable : EnablePort
  ASCII to String : ASCIIToString
  ASCII to String1 : ASCIIToString
  ASCII to String2 : ASCIIToString
  Data Type Conversion1 : DataTypeConversion  OutDataTypeStr=boolean  SaturateOnIntegerOverflow=off  RndMeth=Floor
  String to Double : ScanString  Format="\"%lf\""
  String to Double1 : ScanString  Format="\"%lf\""
  String to Double2 : ScanString  Format="\"%lf\""
  port0_ci_ev_isolation_errorcode : S-Function  FunctionName=sg_mqtt_client_subscribe_s  Parameters="ClientId,  ConnectionId, Topic, QoS, InitValue, Extended, SampleTime"  SFunctionDeploymentMode=off  EnableBusSupport=off  mask(mqtt_client_subscribe_1){ClientId=parClientId, ConnectionId=parConnectionId, Topic='port0/ci/ev/isolation/errorcode', QoS=0 - at most once, InitValue=zeros(1,24,'uint8'), Extended=off, SampleTime=parSampleTime}
      mask prompts: ClientId "Station ID"; ConnectionId "Connection ID"; QoS "Quality of Service"; InitValue "Init Value"; Extended "Extended Interface"; SampleTime "Sample Time [s]"
      mask help: Speedgoat Driver Block<br>MQTT Client - Subscribe<br><br>&copy; 2007 - 2023, Speedgoat GmbH, <a href="matlab: web('www.speedgoat.com','-browser');">www.speedgoat.com</a>
      mask init:
      | sg_mqtt_client_subscribe_m.runMaskInitialization(ClientId, ConnectionId, Topic, InitValue, Extended);
      mask Help: eval('sg.utils.help.show(''io_main/refentry_mqtt_client_subscribe'');')
      mask TypeOptions QoS: 0 - at most once | 1 - at least once | 2 - exactly once
      mask DialogControl groupParameters Prompt: Parameters
      mask Display: disp('Speedgoat\nMQTT Client\nSubscribe\nStation ID: 0\nConnection ID: 0');
  port0_ci_ev_isolation_ready : speedgoatlib_mqtt/Client/MQTT Client Subscribe  ClientId=parClientId  ConnectionId=parConnectionId  Topic='port0/ci/ev/isolation/ready'  QoS=0 - at most once  InitValue=zeros(1,12,'uint8')  Extended=off  SampleTime=parSampleTime
      settings: SourceProductName=MQTT
  port0_ci_ev_isolation_resssoc : S-Function  FunctionName=sg_mqtt_client_subscribe_s  Parameters="ClientId,  ConnectionId, Topic, QoS, InitValue, Extended, SampleTime"  SFunctionDeploymentMode=off  EnableBusSupport=off  mask(mqtt_client_subscribe_1){ClientId=parClientId, ConnectionId=parConnectionId, Topic='port0/ci/ev/isolation/resssoc', QoS=0 - at most once, InitValue=zeros(1,24,'uint8'), Extended=off, SampleTime=parSampleTime}
      mask prompts: ClientId "Station ID"; ConnectionId "Connection ID"; QoS "Quality of Service"; InitValue "Init Value"; Extended "Extended Interface"; SampleTime "Sample Time [s]"
      mask help: Speedgoat Driver Block<br>MQTT Client - Subscribe<br><br>&copy; 2007 - 2023, Speedgoat GmbH, <a href="matlab: web('www.speedgoat.com','-browser');">www.speedgoat.com</a>
      mask init:
      | sg_mqtt_client_subscribe_m.runMaskInitialization(ClientId, ConnectionId, Topic, InitValue, Extended);
      mask Help: eval('sg.utils.help.show(''io_main/refentry_mqtt_client_subscribe'');')
      mask TypeOptions QoS: 0 - at most once | 1 - at least once | 2 - exactly once
      mask DialogControl groupParameters Prompt: Parameters
      mask Display: disp('Speedgoat\nMQTT Client\nSubscribe\nStation ID: 0\nConnection ID: 0');
  EV Ready : Outport
  EV Errorcode : Outport  Port=2
  EV RESS SOC : Outport  Port=3
  wires:
  port0_ci_ev_isolation_ready/1 -> ASCII to String1/1
  port0_ci_ev_isolation_errorcode/1 -> ASCII to String/1
  ASCII to String/1 -> String to Double1/1
  ASCII to String1/1 -> String to Double/1
  String to Double/1 -> Data Type Conversion1/1
  String to Double1/1 -> EV Errorcode/1
  String to Double2/1 -> EV RESS SOC/1
  ASCII to String2/1 -> String to Double2/1
  port0_ci_ev_isolation_resssoc/1 -> ASCII to String2/1
  Data Type Conversion1/1 -> EV Ready/1

== system speedgoatlib_evse/Blocks by Charge State/EVSE Isolation Read /string compare logic ==
  Input : Inport
  ASCII to String1 : ASCIIToString
  Add : Sum
  Gain : Gain  Gain=2
  String Compare : StringCompare
  String Compare1 : StringCompare
  String Constant : StringConstant  String="\"started\""
  String Constant1 : StringConstant  String="\"finished\""
  Out1 : Outport
  wires:
  Input/1 -> ASCII to String1/1
  Add/1 -> Out1/1
  Gain/1 -> Add/2
  String Compare1/1 -> Gain/1
  String Constant/1 -> String Compare/2
  String Compare/1 -> Add/1
  String Constant1/1 -> String Compare1/2
  ASCII to String1/1 -> String Compare/1, String Compare1/1

== system speedgoatlib_evse/Blocks by Charge State/EVSE Isolation Write /Enabled Subsystem ==
  evseprocessing : Inport
  isolationstatus : Inport  Port=2
  statuscode : Inport  Port=3
  Enable : EnablePort
  Constant : Constant  Value=parEnIsolationStatus  OutDataTypeStr=boolean
  Constant1 : Constant  Value=parEnStatusCode  OutDataTypeStr=boolean
  Constant12 : Constant  Value=parEnEvseProcessing  OutDataTypeStr=boolean
  Data Type Conversion1 : DataTypeConversion  OutDataTypeStr=double  SaturateOnIntegerOverflow=off  RndMeth=Floor
  Data Type Conversion3 : DataTypeConversion  OutDataTypeStr=double  SaturateOnIntegerOverflow=off  RndMeth=Floor
  Data Type Conversion4 : DataTypeConversion  OutDataTypeStr=double  SaturateOnIntegerOverflow=off  RndMeth=Floor
  Ground : Ground
  Ground1 : Ground
  Ground12 : Ground
  String to ASCII1 : StringToASCII  OutputVectorSize=12
  String to ASCII2 : StringToASCII  OutputVectorSize=12
  String to ASCII3 : StringToASCII  OutputVectorSize=12
  To String1 : ToString
  To String2 : ToString
  To String3 : ToString
  port0_ci_evse_isolation_evseprocessing : speedgoatlib_mqtt/Client/MQTT Client Publish  ClientId=parClientId  ConnectionId=parConnectionId  Topic='port0/ci/evse/isolation/evseprocessing'  QoS=0 - at most once  Retain=on  Extended=on  SampleTime=parSampleTime
      settings: SourceProductName=MQTT
  port0_ci_evse_isolation_isolationstatus : speedgoatlib_mqtt/Client/MQTT Client Publish  ClientId=parClientId  ConnectionId=parConnectionId  Topic='port0/ci/evse/isolation/isolationstatus'  QoS=0 - at most once  Retain=on  Extended=on  SampleTime=parSampleTime
      settings: SourceProductName=MQTT
  port0_ci_evse_isolation_statuscode : speedgoatlib_mqtt/Client/MQTT Client Publish  ClientId=parClientId  ConnectionId=parConnectionId  Topic='port0/ci/evse/isolation/statuscode'  QoS=0 - at most once  Retain=on  Extended=on  SampleTime=parSampleTime
      settings: SourceProductName=MQTT
  wires:
  Ground1/1 -> port0_ci_evse_isolation_statuscode/3
  Constant1/1 -> port0_ci_evse_isolation_statuscode/2
  Constant/1 -> port0_ci_evse_isolation_isolationstatus/2
  Ground/1 -> port0_ci_evse_isolation_isolationstatus/3
  statuscode/1 -> Data Type Conversion4/1
  isolationstatus/1 -> Data Type Conversion3/1
  String to ASCII2/1 -> port0_ci_evse_isolation_statuscode/1
  String to ASCII1/1 -> port0_ci_evse_isolation_isolationstatus/1
  Data Type Conversion3/1 -> To String1/1
  To String1/1 -> String to ASCII1/1
  To String2/1 -> String to ASCII2/1
  Data Type Conversion4/1 -> To String2/1
  Data Type Conversion1/1 -> To String3/1
  Ground12/1 -> port0_ci_evse_isolation_evseprocessing/3
  Constant12/1 -> port0_ci_evse_isolation_evseprocessing/2
  String to ASCII3/1 -> port0_ci_evse_isolation_evseprocessing/1
  To String3/1 -> String to ASCII3/1
  evseprocessing/1 -> Data Type Conversion1/1

== system speedgoatlib_evse/Blocks by Charge State/EVSE Isolation Write /string compare logic ==
  Input : Inport
  ASCII to String1 : ASCIIToString
  Add : Sum
  Gain : Gain  Gain=2
  String Compare : StringCompare
  String Compare1 : StringCompare
  String Constant : StringConstant  String="\"started\""
  String Constant1 : StringConstant  String="\"finished\""
  Out1 : Outport
  wires:
  Input/1 -> ASCII to String1/1
  Add/1 -> Out1/1
  Gain/1 -> Add/2
  String Compare1/1 -> Gain/1
  String Constant/1 -> String Compare/2
  String Compare/1 -> Add/1
  String Constant1/1 -> String Compare1/2
  ASCII to String1/1 -> String Compare/1, String Compare1/1
